simulink model "MultiRobotDistributedSystem"  (R2024a)
settings: Solver=VariableStepAuto  StartTime=0.0  StopTime=10.0  RelTol=1e-3
undefined symbols (not defined in the file or in its folder): Agents, createNetwork, entity, Tasks
settings Model: Creator=Ryan  LastModifiedBy=Ryan

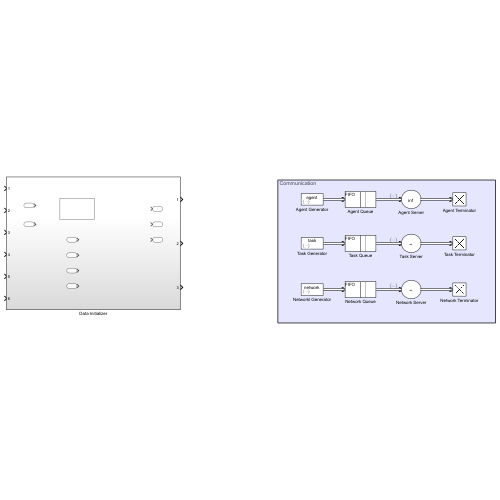
[thumbnail: Simulink's stored preview of the top-level diagram]
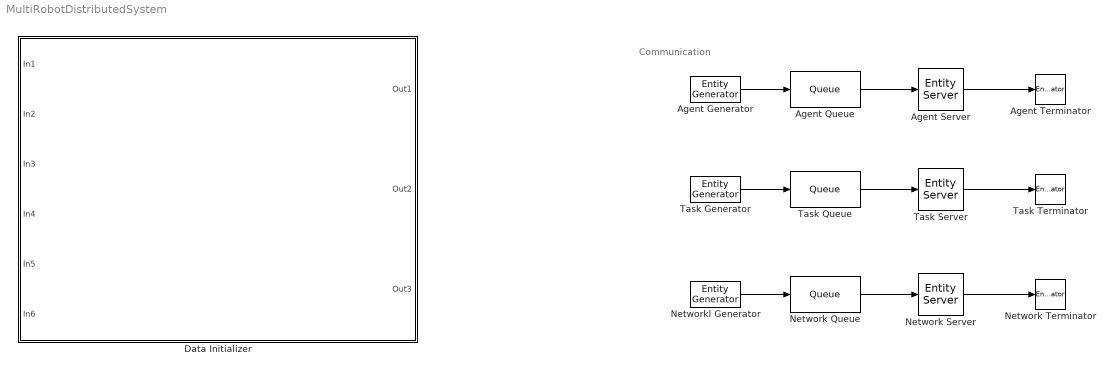
== system MultiRobotDistributedSystem ==
  note: Communication
  Agent Generator : EntityGenerator  OutputPortMessageModes=m  TimeSource=MATLAB action  IntergenerationTimeAction=|  GenerateAction=|  EntityType=Bus object  EntityTypeName=agent
      IntergenerationTimeAction=|
      | persistent dtArray index 
      | if isempty(dtArray)
      |     dtArray = [zeros(1,numAgents-1] inf];
      |     inden = 1;
      | end
      | dt = dtArray(index);
      | index = index + 1;
      GenerateAction=|
      | persistent count
      | if isempty(count)
      |     count = 0;
      | end
      | count = count + 1;
      | entity.Id = count;
      | entity.CurrentPosition = [chargingStations(count,:)';0];
      | entity.Type = AgentType.WarehouseRobot;
      | entity.Footprint = agentFootprint;
  Agent Queue : Queue  InputPortMessageModes=m  OutputPortMessageModes=m  Capacity=inf
  Agent Server : EntityServer  InputPortMessageModes=m  OutputPortMessageModes=m  Capacity=inf  ServiceTimeValue=0.5  EntryAction=Agents.createAgent(entity.Id,entity.CurrentPosition,entity.Type,entity.Foorprint)
  Agent Terminator : EntityTerminator  InputPortMessageModes=m
  Data Initializer : Subsystem
  Network Queue : Queue  InputPortMessageModes=m  OutputPortMessageModes=m  Capacity=inf
  Network Server : EntityServer  InputPortMessageModes=m  OutputPortMessageModes=m  Capacity=inf  ServiceTimeValue=0.5  EntryAction=createNetwork(entity.Map)
  Network Terminator : EntityTerminator  InputPortMessageModes=m
  Networkl Generator : EntityGenerator  OutputPortMessageModes=m  TimeSource=MATLAB action  IntergenerationTimeAction=|  GenerateAction=|  EntityType=Bus object  EntityTypeName=network
      IntergenerationTimeAction=|
      | persistent dtArray index 
      | if isempty(dtArray)
      |     dtArray = [zeros(1,numAgents-1] inf];
      |     inden = 1;
      | end
      | dt = dtArray(index);
      | index = index + 1;
      GenerateAction=|
      | % Pick Maixmum agent radius
      | agentRadius = ceil(sqrt(agentFootprint(1)^2+agentFootprint(2)^2)/2*paddingFactor);
      | for ii = 1:size(logical,1)
      |     for jj = 1:size(logicalMap,2)
      |         entity.Map(ii,jj).Name = [ii;jj]-1;
      |         nodesX = jj - agentRadius:jj+agentRadius-1;
      |         nodesY = size(logcialMap,1)-ii+2-agentRadius:size(logicalMap-1)-ii+1+agentRadius;
      |         if any(nodesY <1)||any(nodesY > size(logicalMap,2)) ||any(nodesX <1)||any(nodesX > size(logicalMap,1))
      |             entity.Map(ii,jj).North = false;
      |             entity.Map(ii,jj).East = false;
      |             entity.Map(ii,jj).West = false;
      |             entity.Map(ii,jj).South = false;
      |         else
      |             open = true;
      |             for kk = 1:length(nodesX)
      |                 for nn = 1:length(nodesY)
      |                     open = open && ~logicalMap(nodesY(nn),nodesX(kk));
      |                 end
      |             end
      |             entity.Map(ii,jj).North = open;
      |             entity.Map(ii,jj).East = open;
      |             entity.Map(ii,jj).South = open;
      |             entity.Map(ii,jj).West = open;
      |         end
      |     end
      | end
      | for ii = 1:size(logicalMap,1)
      |     for jj = 1:size(logicalMap,2)
      |         if ii == 1 || ~entity.Map(ii-1,jj).East
      |             entity.Map(ii,jj).West = false;
      |         end
      |         if ii == size(logicalMap,1) || ~entity.Map(ii+1,jj).West
      |             entity.Map(ii,jj).East = false;
      |         end
      |         if jj == 1|| ~entity.Map(ii,jj-1).North
      |             entity.Map(ii,jj).South = false;
      |         end
      |         if jj == size(logicalMap,2) || ~entity.Map(ii,jj+1).South
      |             entity.Map(ii,jj).North = false;
      |         end
      |     end
      | end
  Task Generator : EntityGenerator  OutputPortMessageModes=m  TimeSource=MATLAB action  IntergenerationTimeAction=|  GenerateAction=|  EntityType=Bus object  EntityTypeName=task
      IntergenerationTimeAction=|
      | persistent dtArray index 
      | if isempty(dtArray)
      |     dtArray = [zeros(1,numAgents-1] inf];
      |     inden = 1;
      | end
      | dt = dtArray(index);
      | index = index + 1;
      GenerateAction=|
      | persistent count
      | if isempty(count)
      |     count = 0;
      | end
      | count = count + 1;
      | entity.Id = count;
      | m = length(loadingStations(:,2);
      | n = length(unloadingStations(:,2);
      | 
      | if (m>1)
      |     entity.Source = loadingStations(packages(count),:)';
      | else
      |     entity.Source = loadingStations(1,:)';
      | end
      | 
      | if(n>1)
      |     entity.Sink = unloadingStations(packages(count),:)';
      | else
      |     entity.Sink = unloadingStations(1,:)';
      | end
  Task Queue : Queue  InputPortMessageModes=m  OutputPortMessageModes=m  Capacity=inf
  Task Server : EntityServer  InputPortMessageModes=m  OutputPortMessageModes=m  Capacity=inf  ServiceTimeValue=0.5  EntryAction=Tasks.createTask(entity.Id,entity.Source,entity.Sink)
  Task Terminator : EntityTerminator  InputPortMessageModes=m
  wires:
  Agent Generator/1 -> Agent Queue/1
  Agent Queue/1 -> Agent Server/1
  Agent Server/1 -> Agent Terminator/1
  Task Queue/1 -> Task Server/1
  Task Server/1 -> Task Terminator/1
  Task Generator/1 -> Task Queue/1
  Network Queue/1 -> Network Server/1
  Network Server/1 -> Network Terminator/1
  Networkl Generator/1 -> Network Queue/1

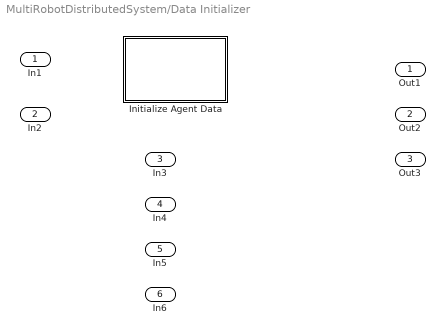
== system MultiRobotDistributedSystem/Data Initializer ==
  In1 : Inport
  In2 : Inport  Port=2
  In3 : Inport  Port=3
  In4 : Inport  Port=4
  In5 : Inport  Port=5
  In6 : Inport  Port=6
  Initialize Agent Data : Subsystem
  Out1 : Outport
  Out2 : Outport  Port=2
  Out3 : Outport  Port=3

== system MultiRobotDistributedSystem/Data Initializer/Initialize Agent Data ==
